simulink model "block_nonlinear_compare"  (R2018a)
settings: Solver=VariableStepAuto  StartTime=0.0  StopTime=10.0  RelTol=1e-3
values from neighbouring files (symbols this model uses):
  den = [1 5]    [SI_Ho_Kalman.m]    (also in SI_MOESP.m; SI_N4SID.m; SVD_identification.m = [1 3]; matrix_test.m = [4 5 6])
  g = v_vals(5)    [Drone_SysId_2step.m]    (also in Drone_System.m; Drone_System_control.m; Drone_System_full.m; Drone_System_identification.m)
  Ix = v_vals(1)    [Drone_SysId_2step.m]    (also in Drone_System.m; Drone_System_control.m; Drone_System_full.m; Drone_System_identification.m)
  Iy = v_vals(2)    [Drone_SysId_2step.m]    (also in Drone_System.m; Drone_System_control.m; Drone_System_full.m; Drone_System_identification.m)
  Iz = v_vals(3)    [Drone_SysId_2step.m]    (also in Drone_System.m; Drone_System_control.m; Drone_System_full.m; Drone_System_identification.m)
  m = v_vals(4)    [Drone_SysId_2step.m]    (also in Drone_System.m = 1; Drone_System_control.m; Drone_System_full.m = 1; Drone_System_identification.m)
  num = [1]    [SI_Ho_Kalman.m]    (also in SI_MOESP.m; SI_N4SID.m; SVD_identification.m; matrix_test.m)
settings Model: Creator=ros  LastModifiedBy=ros

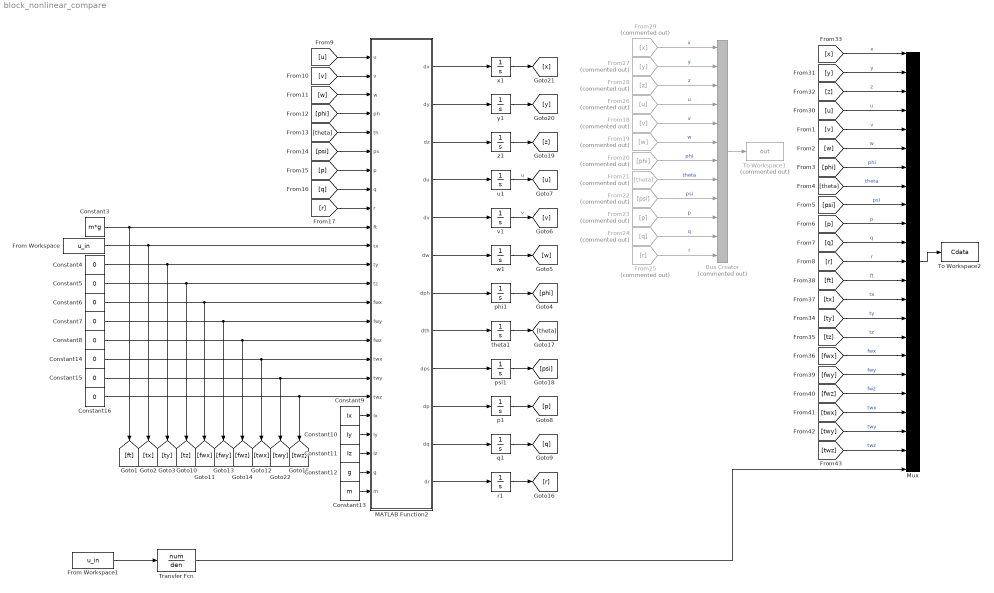
== system block_nonlinear_compare ==
  Bus Creator : BusCreator  Commented=on  Inputs=12
  Constant10 : Constant  Value=Iy
  Constant11 : Constant  Value=Iz
  Constant12 : Constant  Value=g
  Constant13 : Constant  Value=m
  Constant{4..8,14..16} (8 alike) : Constant  Value=0
  Constant3 : Constant  Value=m*g
  Constant9 : Constant  Value=Ix
  From Workspace : FromWorkspace  VariableName=u_in  SampleTime=0.001
  From Workspace1 : FromWorkspace  VariableName=u_in  SampleTime=0.001
  From18 : From  Commented=on  GotoTag=v
  From19 : From  Commented=on  GotoTag=w
  From20 : From  Commented=on  GotoTag=phi
  From21 : From  Commented=on  GotoTag=theta
  From22 : From  Commented=on  GotoTag=psi
  From23 : From  Commented=on  GotoTag=p
  From24 : From  Commented=on  GotoTag=q
  From25 : From  Commented=on  GotoTag=r
  From26 : From  Commented=on  GotoTag=u
  From27 : From  Commented=on  GotoTag=y
  From28 : From  Commented=on  GotoTag=z
  From29 : From  Commented=on  GotoTag=x
  MATLAB Function2 : MATLAB Function  TreatAsAtomicUnit=on
  Mux : Mux  Inputs=23
  To Workspace1 : ToWorkspace  Commented=on  VariableName=out  SaveFormat=Timeseries  SampleTime=-1
  To Workspace2 : ToWorkspace  VariableName=Cdata  SaveFormat=Timeseries  SampleTime=-1
  Transfer Fcn : TransferFcn  Numerator=num  Denominator=den
  p1 : Integrator
  phi1 : Integrator
  psi1 : Integrator
  q1 : Integrator
  r1 : Integrator
  theta1 : Integrator
  u1 : Integrator
  v1 : Integrator
  w1 : Integrator
  x1 : Integrator
  y1 : Integrator
  z1 : Integrator
  wires:
  [v] -> MATLAB Function2/2(v)
  MATLAB Function2/9(dps) -> psi1/1
  MATLAB Function2/10(dp) -> p1/1
  MATLAB Function2/5(dv) -> v1/1
  [r] -> MATLAB Function2/9(r)
  [psi] -> MATLAB Function2/6(ps)
  Constant3/1 -> [ft], MATLAB Function2/10(ft)
  [p] -> MATLAB Function2/7(p)
  p1/1 -> [p]
  MATLAB Function2/12(dr) -> r1/1
  theta1/1 -> [theta]
  [w] -> MATLAB Function2/3(w)
  [phi] -> MATLAB Function2/4(ph)
  [q] -> MATLAB Function2/8(q)
  r1/1 -> [r]
  q1/1 -> [q]
  MATLAB Function2/11(dq) -> q1/1
  phi1/1 -> [phi]
  MATLAB Function2/6(dw) -> w1/1
  MATLAB Function2/4(du) -> u1/1
  psi1/1 -> [psi]
  [u] -> MATLAB Function2/1(u)
  MATLAB Function2/8(dth) -> theta1/1
  [theta] -> MATLAB Function2/5(th)
  u1/1 -> [u]  "u"
  w1/1 -> [w]
  MATLAB Function2/7(dph) -> phi1/1
  v1/1 -> [v]  "v"
  Constant9/1 -> MATLAB Function2/20(Ix)
  Constant13/1 -> MATLAB Function2/24(m)
  Constant11/1 -> MATLAB Function2/22(Iz)
  Constant10/1 -> MATLAB Function2/21(Iy)
  Constant12/1 -> MATLAB Function2/23(g)
  MATLAB Function2/1(dx) -> x1/1
  MATLAB Function2/2(dy) -> y1/1
  MATLAB Function2/3(dz) -> z1/1
  Constant6/1 -> [fwx], MATLAB Function2/14(fwx)
  Constant5/1 -> [tz], MATLAB Function2/13(tz)
  Constant4/1 -> [ty], MATLAB Function2/12(ty)
  Constant7/1 -> [fwy], MATLAB Function2/15(fwy)
  Constant14/1 -> [twx], MATLAB Function2/17(twx)
  Constant8/1 -> [fwz], MATLAB Function2/16(fwz)
  Constant15/1 -> [twy], MATLAB Function2/18(twy)
  Constant16/1 -> [twz], MATLAB Function2/19(twz)
  Bus Creator/1 -> To Workspace1/1
  z1/1 -> [z]
  y1/1 -> [y]
  x1/1 -> [x]
  From29/1 -> Bus Creator/1  "x"
  From27/1 -> Bus Creator/2  "y"
  From28/1 -> Bus Creator/3  "z"
  From26/1 -> Bus Creator/4  "u"
  From18/1 -> Bus Creator/5  "v"
  From19/1 -> Bus Creator/6  "w"
  From20/1 -> Bus Creator/7  "phi"
  From21/1 -> Bus Creator/8  "theta"
  From22/1 -> Bus Creator/9  "psi"
  From23/1 -> Bus Creator/10  "p"
  From24/1 -> Bus Creator/11  "q"
  From25/1 -> Bus Creator/12  "r"
  From Workspace/1 -> [tx], MATLAB Function2/11(tx)
  [x] -> Mux/1  "x"
  [v] -> Mux/5  "v"
  [z] -> Mux/3  "z"
  [w] -> Mux/6  "w"
  [p] -> Mux/10  "p"
  [phi] -> Mux/7  "phi"
  [theta] -> Mux/8  "theta"
  [r] -> Mux/12  "r"
  [y] -> Mux/2  "y"
  [psi] -> Mux/9  "psi"
  [u] -> Mux/4  "u"
  [q] -> Mux/11  "q"
  Mux/1 -> To Workspace2/1
  [ft] -> Mux/13  "ft"
  [tx] -> Mux/14  "tx"
  [ty] -> Mux/15  "ty"
  [tz] -> Mux/16  "tz"
  [fwx] -> Mux/17  "fwx"
  [fwy] -> Mux/18  "fwy"
  [fwz] -> Mux/19  "fwz"
  [twx] -> Mux/20  "twx"
  [twy] -> Mux/21  "twy"
  [twz] -> Mux/22  "twz"
  From Workspace1/1 -> Transfer Fcn/1
  Transfer Fcn/1 -> Mux/23

== matlab function block_nonlinear_compare/MATLAB Function2 ==
  data: u input; v input; dx output; w input; ph input; th input; ps input; p input; q input; r input; ft input; tx input; ty input; tz input; fwx input; fwy input; fwz input; twx input; twy input; twz input; dy output; dz output; du output; dv output; dw output; dph output; dth output; dps output; dp output; dq output; dr output; Ix input; Iy input; Iz input; g input; m input
function [dx, dy, dz, du, dv, dw, dph, dth, dps, dp, dq, dr] = fcn(u, v, w, ph, th, ps, p, q, r, ft, tx, ty, tz, fwx, fwy, fwz, twx, twy, twz, Ix, Iy, Iz, g, m)

dx = w*(sin(ph)*sin(ps) + cos(ph)*cos(ps)*sin(th)) - v*(cos(ph)*sin(ps) - cos(ps)*sin(ph)*sin(th)) + u*(cos(ps)*cos(th));
dy = v*(cos(ph)*cos(ps) + sin(ph)*sin(ps)*sin(th)) - w*(cos(ps)*sin(ph) - cos(ph)*sin(ps)*sin(th)) + u*(cos(th)*sin(ps));
dz = w*(cos(ph)*cos(th)) - u*(sin(th)) + v*(cos(th)*sin(ph));
du = r*v - q*w + g*(sin(th)) + fwx / m;
dv = p*w - r*u - g*(sin(ph)*cos(th)) + fwy / m;
dw = q*u - p*v - g*(cos(th)*cos(ph)) + (fwz + ft) / m;
dph = p + r*(cos(ph)*tan(th)) + q*(sin(ph)*tan(th));
dth = q*(cos(th)) - r*(sin(ph));
dps = r*(cos(ph)/cos(th)) + q*(sin(ph)/cos(th));
dp = r*q*(Iy - Iz)/Ix + (tx + twx)/Ix;
dq = p*r*(Iz - Ix)/Iy + (ty + twy)/Iy;
dr = p*q*(Ix - Iy)/Iz + (tz + twz)/Iz;
